simulink model "HelloWorld"  (R2017a)
settings: Solver=FixedStepDiscrete  StartTime=0.0  StopTime=inf  FixedStep=0.01  RelTol=1e-3
settings Model: Creator=ashish  LastModifiedBy=ashish
settings HardwareCC: ProdBitPerPointer=32  ProdBitPerSizeT=32  ProdBitPerPtrDiffT=32  ProdLargestAtomicInteger=Long  ProdLargestAtomicFloat=Double  ProdWordSize=32  ProdHWDeviceType=ARM Compatible->ARM Cortex

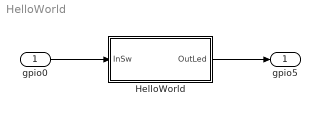
== system HelloWorld ==
  gpio0 : Inport
  HelloWorld : Subsystem  TreatAsAtomicUnit=on
  gpio5 : Outport
  wires:
  HelloWorld/1(OutLed) -> gpio5/1
  gpio0/1 -> HelloWorld/1(InSw)

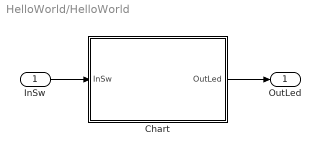
== system HelloWorld/HelloWorld ==
  InSw : Inport
  Chart : Stateflow chart  TreatAsAtomicUnit=on
  OutLed : Outport
  wires:
  InSw/1 -> Chart/1(InSw)
  Chart/1(OutLed) -> OutLed/1

== stateflow chart HelloWorld/Chart ==
  state LedBlinkWithConsolePrint
    state SerialPrint [parallel]
      /* This state prints on the console */
      settings: executionOrder=2
      (default) -> (junction 9)
      SerialPrint -> (junction 9)
      (junction 9) -> (junction 13) [order 1] : [ count1 > 1000000]
      (junction 13) -> (junction 12) : {
          |  count1 = 0;
          |  count2++;
          |  printf("Execution timer has incremented by %d\n", count2);
          | }
      (junction 9) -> (junction 12) [order 2] : {
          |  count1++;
          | }
    state LedOut [parallel]
      /* This state reads the input switch and turns off or on the Led */
      settings: executionOrder=1
      state On
        /*Turn the led on*/
        en,du:
        OutLed = 1;
      state Off
        /* Keep the led off */
        en,du:
        OutLed = 0;
      (default) -> Off
      Off -> On : [InSw == 1]
      On -> Off : [InSw == 0]
  (default) -> LedBlinkWithConsolePrint
  data: InSw input; OutLed output; count1 local uint32; count2 local uint32
